simulink model "pathfollower"  (R2013a)
settings: Solver=ode3  SolverMode=SingleTasking  StartTime=0.0  StopTime=inf  RelTol=1e-3
libraries: legonxtlib x2
settings Model: SimulationMode=external  ExtModeTrigDuration=2  Creator=anton  LastModifiedBy=anton
settings OptimizationCC: OptimizeModelRefInitCode=on  LifeSpan=1
settings DebuggingCC: SolverPrmCheckMsg=none  StrictBusMsg=Warning
settings HardwareCC: ProdLargestAtomicInteger=Long  ProdLargestAtomicFloat=Float  ProdEndianess=LittleEndian  ProdHWDeviceType=ARM Compatible->ARM 7
settings RTWCC: SystemTargetFile=realtime.tlc  GenerateMakefile=off  TemplateMakefile=realtime.tmf  Description=Run on Target Hardware  RTWVerbose=off  ProcessScript=realtime_make_rtw_hook
settings STFCustomTargetCC: TargetLibSuffix=.a  GenerateSampleERTMain=on  ERTCustomFileBanners=on  SupportNonInlinedSFcns=off  SupportVariableSizeSignals=on  MATLABClassNameForMDSCustomization=Simulink.SoftwareTarget.ERTCustomization  SystemTargetFile=realtime.tlc
settings ERTTargetCC: ParMdlRefBuildCompliant=off  CompOptLevelCompliant=off  ConcurrentExecutionCompliant=off  CombineOutputUpdateFcns=off  ERTFirstTimeCompliant=off  SupportContinuousTime=on  SupportVariableSizeSignals=on  ModelStepFunctionPrototypeControlCompliant=off  CPPClassGenCompliant=off  ExtMode=on  ExtModeTransport=2  ExtModeMexFile=ext_serial_win32_comm_no_acks_rtt  ExtModeMexArgs=0 5 9600  ERTSrcFileBannerTemplate=realtime_code_template.cgt  ERTHdrFileBannerTemplate=realtime_code_template.cgt  ERTDataSrcFileTemplate=realtime_code_template.cgt  ERTDataHdrFileTemplate=realtime_code_template.cgt  ERTCustomFileTemplate=realtime_file_process.tlc

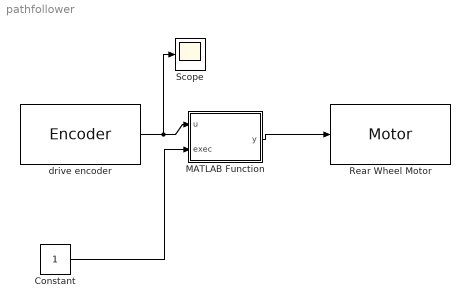
== system pathfollower ==
  Constant : Constant
  MATLAB Function : MATLAB Function  TreatAsAtomicUnit=on
  Rear Wheel Motor : legonxtlib/Motor  sportNumber=C  sstopAction=Brake
  Scope : Scope
      settings: YMin=3570  YMax=3570
  drive encoder : legonxtlib/Encoder  portNumber=C  opMode=No reset  sampleTime=0.1
  wires:
  MATLAB Function/1(y) -> Rear Wheel Motor/1
  drive encoder/1 -> Scope/1, MATLAB Function/1(u)
  Constant/1 -> MATLAB Function/2(exec)

== matlab function pathfollower/MATLAB Function ==
  data: u input; y output; exec input
function y = fcn(u,exec)
%#codegen
radius = 2.5/100;
circ = radius*2*pi;

if exec == 1
    if u < 3000
        y = 15;
    else
        y = 0;
    end
else
    y = 0;
end
